simulink model "HWC"  (R2018a)
settings: Solver=FixedStepAuto  StartTime=0.0  StopTime=stopTime  FixedStep=stepSize  RelTol=1e-3
values from neighbouring files (symbols this model uses):
  n = n_D    [AA279D_hw4.m]    (also in AA279D_hw4_v2.m = sqrt(mu/a^3); AA279D_hw5_dv.m = sqrt(mu/at^3); OE2ECI.m = sqrt(mu/a^3); TLE_Reader.m = revs_per_day*2*pi/(24*3600))
  rho_RTN_init = T_ECI2RTN*(r2_ECI_init-r_ECI_init)    [AA279D_PSET2.m]    (also in AA279D_PSET2_a_change.m; AA279D_PSET3.m; AA279D_PSET4.m; AA279D_hw4_v2.m)
  rhod_RTN_init = T_ECI2RTN*(v2_ECI_init-v_ECI_init)-     cross([0;0;thd0],rho_RTN_init)    [AA279D_PSET2.m]    (also in AA279D_PSET2_a_change.m; AA279D_PSET3.m; AA279D_PSET4.m; AA279D_hw4_v2.m)
  stepSize = 5    [AA279D_FINAL.m]    (also in AA279D_PSET1.m = 1; AA279D_PSET2.m; AA279D_PSET2_a_change.m = 1; AA279D_PSET3.m)
settings Model: Creator=Christopher Covert  LastModifiedBy=Christopher Covert

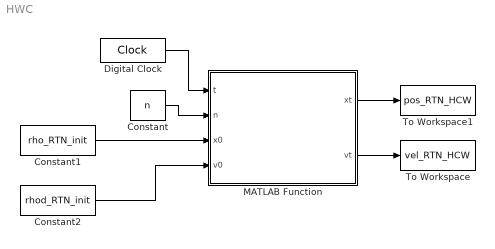
== system HWC ==
  Constant : Constant  Value=n
  Constant1 : Constant  Value=rho_RTN_init
  Constant2 : Constant  Value=rhod_RTN_init
  Digital Clock : DigitalClock  SampleTime=stepSize
  MATLAB Function : MATLAB Function  TreatAsAtomicUnit=on
  To Workspace : ToWorkspace  VariableName=vel_RTN_HCW  SampleTime=-1
  To Workspace1 : ToWorkspace  VariableName=pos_RTN_HCW  SampleTime=-1
  wires:
  Constant/1 -> MATLAB Function/2(n)
  MATLAB Function/1(xt) -> To Workspace1/1
  MATLAB Function/2(vt) -> To Workspace/1
  Constant1/1 -> MATLAB Function/3(x0)
  Constant2/1 -> MATLAB Function/4(v0)
  Digital Clock/1 -> MATLAB Function/1(t)

== matlab function HWC/MATLAB Function ==
  data: t input; n input; xt output; x0 input; v0 input; vt output
function [xt,vt] = HCW_PROP(t,n,x0,v0)

x = x0(1); dx = v0(1);
y = x0(2); dy = v0(2);
z = x0(3); dz = v0(3);

s = sin(n*t);
c = cos(n*t);

eAt = [1 0 -c s 0 0;
    -1.5*t 1 2*s -2*c 0 0;
    0 0 0 0 s -c;
    0 0 s -c 0 0;
    -1.5 0 2*c 2*s 0 0;
    0 0 0 0 c s];

x_all = eAt*x0;


xt = x_all(1:3);
vt = x_all(4:6);

end
